simulink model "s_tanks_1"  (Simulink 7.0)
settings: Solver=ode4  StartTime=0.0  StopTime=60  FixedStep=0.002  RelTol=1e-3
undefined symbols (not defined in the file or in its folder): Ao1, At1, g, Kff_1, Ki_1, Kp, Kp_1, L10, MAX_L1_WDUP, TS, VMAX_AMP
settings Model: Creator=MLevis  LastModifiedBy=aabdossalami  ExtModeTrigDuration=30000
settings SolverCC: PositivePriorityOrder=on
settings DebuggingCC: SaveWithParameterizedLinksMsg=none
settings RTWCC: SystemTargetFile=quarc_windows.tlc  TemplateMakefile=quarc_default_tmf  Description=QuaRC Win32 Target  ProcessScript=quarc_windows_make_rtw_hook
settings STFCustomTargetCC: TargetFcnLib=ansi_tfl_tmw.mat  TargetPreCompLibLocation=C:\DOCUME~1\ALLUSE~1\APPLIC~1\QUARC\lib\2007b\windows\release  GenFloatMathFcnCalls=ANSI_C  SystemTargetFile=quarc_windows.tlc
settings GRTTargetCC: TargetFcnLib=ansi_tfl_tmw.mat  TargetPreCompLibLocation=C:\DOCUME~1\ALLUSE~1\APPLIC~1\QUARC\lib\2007b\windows\release  CompOptLevelCompliant=off  MatFileLogging=off  ExtMode=on  ExtModeMexFile=quarc_comm

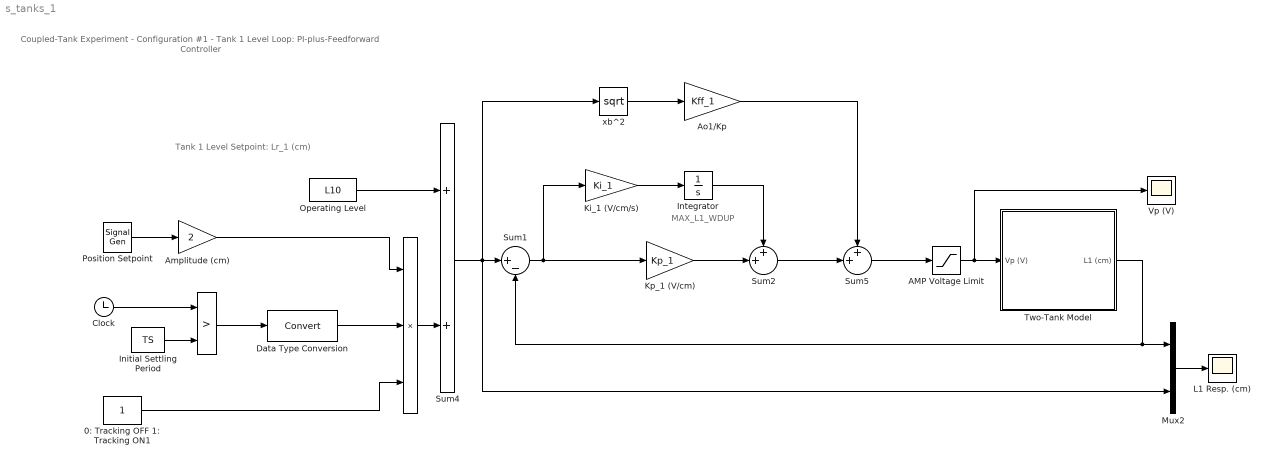
== system s_tanks_1 ==
  note: Coupled-Tank Experiment
      | - Configuration #1 -
      | Tank 1 Level Loop:
      | PI-plus-Feedforward Controller
  note: Tank 1 Level Setpoint:
      | Lr_1 (cm)
  note: MAX_L1_WDUP
  "   " : Product  Inputs=3  OutDataType=sfix(16)  OutScaling=2^0  SaturateOnIntegerOverflow=on  RndMeth=Zero  InputSameDT=on
  "    " : RelationalOperator  Operator=>  InputSameDT=on
  0: Tracking OFF 1: Tracking ON1 : Constant  OutDataType=sfix(16)  OutScaling=2^0
  AMP Voltage Limit : Saturate  UpperLimit=VMAX_AMP  LowerLimit=0
  Amplitude (cm) : Gain  Gain=2  ParameterDataType=sfix(16)  ParameterScaling=2^0  OutDataType=sfix(16)  OutScaling=2^0  SaturateOnIntegerOverflow=on
  Ao1/Kp : Gain  Gain=Kff_1  ParameterDataType=sfix(16)  ParameterScaling=2^0  OutDataType=sfix(16)  OutScaling=2^0  SaturateOnIntegerOverflow=on
  Clock : Clock
      settings: Decimation=10
  Data Type Conversion : DataTypeConversion  OutDataType=sfix(16)  OutScaling=2^0
  Initial Settling Period : Constant  Value=TS  OutDataType=sfix(16)  OutScaling=2^0
  Integrator : Integrator  LimitOutput=on  UpperSaturationLimit=MAX_L1_WDUP  LowerSaturationLimit=- MAX_L1_WDUP
  Ki_1 (V/cm/s) : Gain  Gain=Ki_1  ParameterDataType=sfix(16)  ParameterScaling=2^0  OutDataType=sfix(16)  OutScaling=2^0  SaturateOnIntegerOverflow=on
  Kp_1 (V/cm) : Gain  Gain=Kp_1  ParameterDataType=sfix(16)  ParameterScaling=2^0  OutDataType=sfix(16)  OutScaling=2^0  SaturateOnIntegerOverflow=on
  L1 Resp. (cm) : Scope
      settings: TickLabels=on  TimeRange=60  YMin=10  YMax=20  SaveName=data_L1  DataFormat=Array
  Mux2 : Mux  Inputs=2
  Operating Level : Constant  Value=L10  OutDataType=sfix(16)  OutScaling=2^0
  Position Setpoint : SignalGenerator  WaveForm=square  Frequency=0.05
  Sum1 : Sum  Inputs=|+-  OutDataType=sfix(16)  OutScaling=2^0  SaturateOnIntegerOverflow=on  InputSameDT=on
  Sum2 : Sum  Inputs=++|  OutDataType=sfix(16)  OutScaling=2^0  SaturateOnIntegerOverflow=on  InputSameDT=on
  Sum4 : Sum  OutDataType=sfix(16)  OutScaling=2^0  SaturateOnIntegerOverflow=on  InputSameDT=on
  Sum5 : Sum  Inputs=++|  OutDataType=sfix(16)  OutScaling=2^0  SaturateOnIntegerOverflow=on  InputSameDT=on
  Two-Tank Model : Subsystem
  "Vp (V) " : Scope
      settings: TickLabels=on  TimeRange=60  YMax=24  SaveName=data_Vp  DataFormat=Array
  xb^2 : Math  Operator=sqrt  OutDataType=sfix(16)  OutScaling=2^0  SaturateOnIntegerOverflow=on
  wires:
  Mux2/1 -> L1 Resp. (cm)/1
  Sum1/1 -> Kp_1 (V/cm)/1, Ki_1 (V/cm/s)/1
  Ki_1 (V/cm/s)/1 -> Integrator/1
  Kp_1 (V/cm)/1 -> Sum2/2
  Integrator/1 -> Sum2/1
  AMP Voltage Limit/1 -> Two-Tank Model/1(Vp (V)), "Vp (V) "/1
  Sum4/1 -> xb^2/1, Sum1/1, Mux2/2
  Sum2/1 -> Sum5/2
  Sum5/1 -> AMP Voltage Limit/1
  xb^2/1 -> Ao1/Kp/1
  Ao1/Kp/1 -> Sum5/1
  Two-Tank Model/1(L1 (cm)) -> Sum1/2, Mux2/1
  Position Setpoint/1 -> Amplitude (cm)/1
  0: Tracking OFF 1: Tracking ON1/1 -> "   "/3
  "   "/1 -> Sum4/2
  Operating Level/1 -> Sum4/1
  Initial Settling Period/1 -> "    "/2
  Clock/1 -> "    "/1
  Amplitude (cm)/1 -> "   "/1
  "    "/1 -> Data Type Conversion/1
  Data Type Conversion/1 -> "   "/2

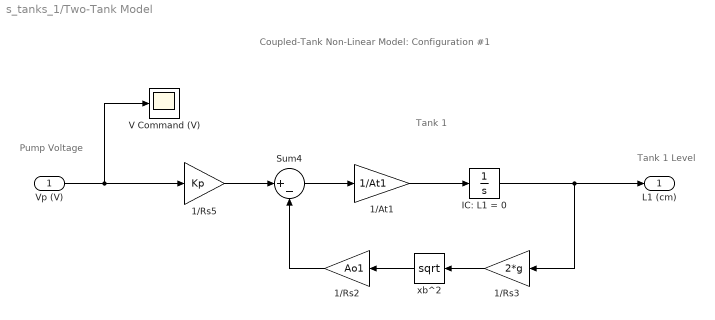
== system s_tanks_1/Two-Tank Model ==
  note: Coupled-Tank Non-Linear Model:
      | Configuration #1
  note: Tank 1
  note: Tank 1 Level
  note: Pump
      | Voltage
  Vp (V) : Inport  OutDataType=sfix(16)  OutScaling=2^0
  1/At1 : Gain  Gain=1/At1  ParameterDataType=sfix(16)  ParameterScaling=2^0  OutDataType=sfix(16)  OutScaling=2^0  SaturateOnIntegerOverflow=on
  1/Rs2 : Gain  Orientation=left  Gain=Ao1  ParameterDataType=sfix(16)  ParameterScaling=2^0  OutDataType=sfix(16)  OutScaling=2^0  SaturateOnIntegerOverflow=on
  1/Rs3 : Gain  Orientation=left  Gain=2*g  ParameterDataType=sfix(16)  ParameterScaling=2^0  OutDataType=sfix(16)  OutScaling=2^0  SaturateOnIntegerOverflow=on
  1/Rs5 : Gain  Gain=Kp  ParameterDataType=sfix(16)  ParameterScaling=2^0  OutDataType=sfix(16)  OutScaling=2^0  SaturateOnIntegerOverflow=on
  IC: L1 = 0 : Integrator
  Sum4 : Sum  Inputs=|+-  OutDataType=sfix(16)  OutScaling=2^0  SaturateOnIntegerOverflow=on  InputSameDT=on
  V Command (V) : Scope
      settings: TickLabels=on  TimeRange=1.000000  YMin=-1  YMax=1  SaveName=ScopeData2  DataFormat=Array
  xb^2 : Math  Orientation=left  Operator=sqrt  OutDataType=sfix(16)  OutScaling=2^0  SaturateOnIntegerOverflow=on
  L1 (cm) : Outport  OutDataType=sfix(16)  OutScaling=2^0  InitialOutput=0
  wires:
  Vp (V)/1 -> V Command (V)/1, 1/Rs5/1
  1/Rs5/1 -> Sum4/1
  Sum4/1 -> 1/At1/1
  1/At1/1 -> IC: L1 = 0/1
  IC: L1 = 0/1 -> 1/Rs3/1, L1 (cm)/1
  1/Rs2/1 -> Sum4/2
  xb^2/1 -> 1/Rs2/1
  1/Rs3/1 -> xb^2/1
